simulink model "Inversores_simu"  (R2024b)
settings: Solver=FixedStepDiscrete  StartTime=0.0  StopTime=10/f  FixedStep=fixed_step  RelTol=1e-3
PostLoadFcn:
  | if any(exist('dsrtsu_mdlpostloadfcn', 'file') ~= 0), dsrtsu_mdlpostloadfcn('Execute', bdroot); end
InitFcn:
  | % Solver
  | fixed_step = 1e-6;
  | sample_time = fixed_step;
  | 
  | % Frecuencia fundamental del inversor
  | f = 60;
undefined symbols (not defined in the file): C
libraries: spsFourierLib x24, spsIGBTDiodeLib x8, spsMultimeterLib x4, spsRMSLib x4, spsTHDLib x4, spsSeriesRLCBranchLib x2, spsTriangleGeneratorLib x2, spsDCVoltageSourceLib x2, spsVoltageMeasurementLib x1, spspowerguiLib x1
settings Model: DSRTSU_INTERNAL_RTI_VER=530  DSRTSU_INTERNAL_RTI_TYPE=rti1202  RTICANMMDATA=struct('GeneralSetupData',struct('modelroot','C:\Users\jjmd2\OneDrive\Escritorio','generalsettings',struct('filesettings',struct('destfolder',struct('Name','RTICANMM_FILES','Check',1),'buildfolder',struct('Name','.','Check',1),'AbsDestfolder',struct('Name','C:\Users\jjmd2\OneDrive\Escritorio\RTICANMM_FILES'),'AbsBuildfolder',struct('Name','C:\Users\jjmd2\OneDrive\Escritorio'))),'options',struct('addpaths',1,'rmpaths',1,'addtrcexclusion',logical(1),'cannavigator',struct('checkmonitoring',0),'show_usrtrc',0,'use_usrtrc',0),'advanced',struct('options',ones(1,100)),'MPSetup',{{}},'RTI',struct('Type','RTI1202','Ver','7.11','Date','02-Nov-2018'),'modelname','libreria_potencia','block','libreria_potencia'))  Creator=jjmd2  LastModifiedBy=PC
settings SolverCC: AlgebraicLoopSolver=TrustRegion
settings OptimizationCC: BlockReduction=off
settings DebuggingCC: UnconnectedInputMsg=warning  UnconnectedOutputMsg=warning  UnconnectedLineMsg=warning
settings HardwareCC: ProdBitPerPointer=32  ProdBitPerSizeT=32  ProdBitPerPtrDiffT=32  ProdLargestAtomicInteger=Integer  ProdEndianess=BigEndian  ProdWordSize=32  ProdHWDeviceType=Custom Processor->Custom  TargetIntDivRoundTo=Zero  TargetEndianess=BigEndian  TargetHWDeviceType=Custom Processor->Custom
settings ModelReferenceCC: EnableRefExpFcnMdlSchedulingChecks=on
settings SFSimCC: MATLABDynamicMemAlloc=off
settings RTWCC: Description=dSPACE DS1202 Hardware Platform  SystemTargetFile=rti1202.tlc  MakeCommand=make_rti  TemplateMakefile=rti1202.tmf  GPUComputeCapability=3.5  DLArmComputeVersion=19.05
settings STFCustomTargetCC: ParMdlRefBuildCompliant=on  SystemTargetFile=rti1202.tlc
settings GRTTargetCC: TargetLangStandard=C89/C90 (ANSI)  CompOptLevelCompliant=off  ConcurrentExecutionCompliant=off  CombineOutputUpdateFcns=off  MatFileLogging=off  CPPClassGenCompliant=off  UseToolchainInfoCompliant=off

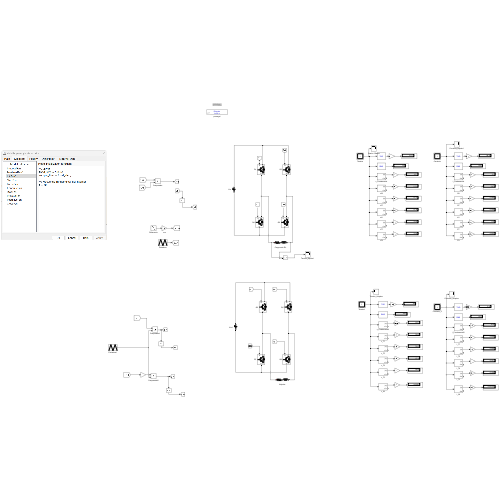
[thumbnail: Simulink's stored preview of the top-level diagram]
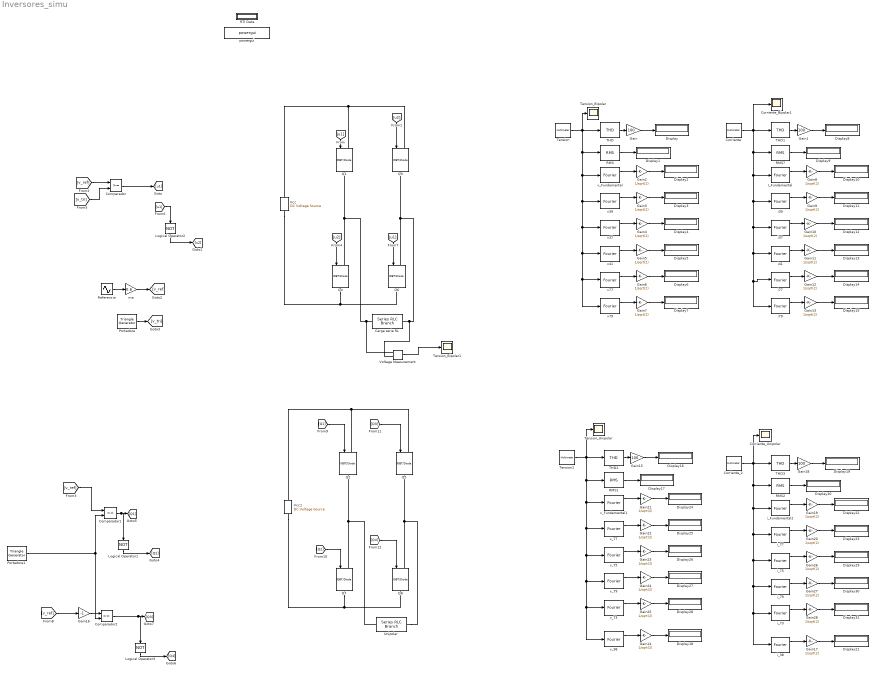
== system Inversores_simu ==
  Carga serie RL : spsSeriesRLCBranchLib/Series RLC Branch  LConnTagsString=__new0  RConnTagsString=__new0  BranchType=RL  Resistance=10  Inductance=5e-3  SetiL0=off  InitialCurrent=0  Capacitance=C  Setx0=off  InitialVoltage=0  Measurements=Branch voltage and current
  Comparador : RelationalOperator  OutDataTypeStr=boolean  RndMeth=Simplest  InputSameDT=off
  Comparador1 : RelationalOperator  OutDataTypeStr=boolean  RndMeth=Simplest  InputSameDT=off
  Comparador2 : RelationalOperator  OutDataTypeStr=boolean  RndMeth=Simplest  InputSameDT=off
  Corriente : spsMultimeterLib/Multimeter  L=4  sel=3  yselected={}  Gain=1  OutputType=Complex  PlotAtSimulationStop=off  PhasorSimulation=off
  Corriente_2 : spsMultimeterLib/Multimeter  L=4  sel=4  yselected={}  Gain=1  OutputType=Complex  PlotAtSimulationStop=off  PhasorSimulation=off
  Corriente_Bipolar1 : Scope
  Corriente_Unipolar : Scope
  Display{,1..31} (32 alike) : Display
  Gain{,1,15,18} (4 alike) : Gain  Gain=100
  Gain{2..14,17,19..28} (24 alike) : Gain  Gain=1/sqrt(2)
  Gain16 : Gain  Gain=-1
  I_Fundamental : spsFourierLib/Fourier  Freq=60  n=1  InInit=[0, 0]  Ts=sample_time
  Logical Operator1 : Logic  Operator=NOT  AllPortsSameDT=off  OutDataTypeStr=boolean
  Logical Operator2 : Logic  Operator=NOT  AllPortsSameDT=off  OutDataTypeStr=boolean
  Logical Operator3 : Logic  Operator=NOT  AllPortsSameDT=off  OutDataTypeStr=boolean
  Portadora : spsTriangleGeneratorLib/Triangle Generator  Freq=39*60  Phase=0  Ts=sample_time
  Portadora1 : spsTriangleGeneratorLib/Triangle Generator  Freq=38*60  Phase=0  Ts=sample_time
  Q{1..8} (8 alike) : spsIGBTDiodeLib/IGBT//Diode  Ron=1e-3  Rs=1000  Cs=0.1e-6  Measurements=off
  RMS{,1..2,7} (4 alike) : spsRMSLib/RMS  TrueRMS=on  Freq=60  RMSInit=120  Ts=sample_time
  RTI Data : Subsystem  Tag=struct('RTIDataServer',struct('RTIDataServerVs','2','RTIModelDescription','struct(''main'',''plantilla_modelos'',''sub'',''plantilla_modelos'',''isMp'',0)'))  LoadFcn="if exist('rtidc'), try,  rtidc('DataHostBlockClbLoad', gcbh); catch, disp(['Warning: ''LoadFcn'' for RTI Data block failed: ' lasterr]); end, end,"  mask(RTI_DATA_HOST){}
      mask help:
      | RTI Data Block.
      | This block is used by RTI to store internal model-dependent data.
      | Please keep this block on the root level of the model. Deleting this block will result in data loss.
      |
      | NEVER DELETE OR COPY THIS BLOCK!
      settings: CopyFcn="if exist('rtidc'), try,  rtidc('DataHostBlockClbCopy', gcbh); catch, disp(['Warning: ''CopyFcn'' for RTI Data block failed: ' lasterr]); end, end,"  DeleteFcn="if exist('rtidc'), try,  rtidc('DataHostBlockClbDelete', gcbh); catch, disp(['Warning: ''DeleteFcn'' for RTI Data block failed: ' lasterr]); end, end,"  ModelCloseFcn="if exist('rtidc'), try,  rtidc('DataHostBlockClbModelClose', gcbh); catch, disp(['Warning: ''ModelCloseFcn'' for RTI Data block failed: ' lasterr]); end, end,"  PreSaveFcn="if exist('rtidc'), try,  rtidc('DataHostBlockClbPreSave', gcbh); catch, disp(['Warning: ''PreSaveFcn'' for RTI Data block failed: ' lasterr]); end, end,"  PostSaveFcn="if exist('rtidc'), try,  rtidc('DataHostBlockClbPostSave', gcbh); catch, disp(['Warning: ''PostSaveFcn'' for RTI Data block failed: ' lasterr]); end, end,"  NameChangeFcn="if exist('rtidc'), try,  rtidc('DataHostBlockClbNameChange', gcbh); catch, disp(['Warning: ''NameChangeFcn'' for RTI Data block failed: ' lasterr]); end, end,"
      mask Help:
      | RTI Data Block.
      | This block is used by RTI to store internal model-dependent data.
      | Please keep this block on the root level of the model. Deleting this block will result in data loss.
      | 
      | NEVER DELETE OR COPY THIS BLOCK!
      mask Display:
      | text(0.5, 0.5, 'RTI Data', 'HorizontalAlignment', 'center');
      | plot([1 0]);
  Referencia : Sin  Frequency=2*pi*f  SampleTime=sample_time
  THD{,1..3} (4 alike) : spsTHDLib/THD  Freq=60  Ts=sample_time
  Tension : spsMultimeterLib/Multimeter  L=4  sel=1  yselected={}  Gain=1  OutputType=Complex  PlotAtSimulationStop=off  PhasorSimulation=off
  Tension1 : spsMultimeterLib/Multimeter  L=4  sel=2  yselected={}  Gain=1  OutputType=Complex  PlotAtSimulationStop=off  PhasorSimulation=off
  Tension_Bipolar : Scope
  Tension_Bipolar1 : Scope
  Tension_Unipolar : Scope
  Unipolar : spsSeriesRLCBranchLib/Series RLC Branch  LConnTagsString=__new0  RConnTagsString=__new0  BranchType=RL  Resistance=10  Inductance=5e-3  SetiL0=off  InitialCurrent=0  Capacitance=C  Setx0=off  InitialVoltage=0  Measurements=Branch voltage and current
  Vcc : spsDCVoltageSourceLib/DC Voltage Source  Amplitude=300  Measurements=None
  Vcc1 : spsDCVoltageSourceLib/DC Voltage Source  Amplitude=300  Measurements=None
  Voltage Measurement : spsVoltageMeasurementLib/Voltage Measurement  PhasorSimulation=off  OutputType=Complex  PSBequivalent=0
  i37 : spsFourierLib/Fourier  Freq=60  n=37  InInit=[0, 0]  Ts=sample_time
  i39 : spsFourierLib/Fourier  Freq=60  n=39  InInit=[0, 0]  Ts=sample_time
  i41 : spsFourierLib/Fourier  Freq=60  n=41  InInit=[0, 0]  Ts=sample_time
  i77 : spsFourierLib/Fourier  Freq=60  n=77  InInit=[0, 0]  Ts=sample_time
  i79 : spsFourierLib/Fourier  Freq=60  n=79  InInit=[0, 0]  Ts=sample_time
  i_38 : spsFourierLib/Fourier  Freq=60  n=38  InInit=[0, 0]  Ts=sample_time
  i_73 : spsFourierLib/Fourier  Freq=60  n=73  InInit=[0, 0]  Ts=sample_time
  i_75 : spsFourierLib/Fourier  Freq=60  n=75  InInit=[0, 0]  Ts=sample_time
  i_77 : spsFourierLib/Fourier  Freq=60  n=77  InInit=[0, 0]  Ts=sample_time
  i_79 : spsFourierLib/Fourier  Freq=60  n=79  InInit=[0, 0]  Ts=sample_time
  i_Fundamental2 : spsFourierLib/Fourier  Freq=60  n=1  InInit=[0, 0]  Ts=sample_time
  ma : Gain  Gain=0.6
  powergui : spspowerguiLib/powergui  Priority=1  SimulationMode=Discrete  SampleTime=sample_time  frequency=60  Iterations=50  frequencyindice=0  Pbase=100e6  ErrMax=1e-4  UnitsV=kV  UnitsW=MW  buscounter=0  FunctionMessages=off  echomessages=off  EnableUseOfTLC=off  CurrentSourceSwitches=off  DisableSnubberDevices=off  DisableRonSwitches=off  DisableVfSwitches=off  DisplayEquations=off  AutomaticDiscreteSolvers=off  SolverType=Tustin/Backward Euler (TBE)  Interpol=off  ExternalGateDelay=off  methode=off  Ts=100  x0status=blocks  SPID=off  SwTol=0  HookPort=off  NonlinearTolerance=1e-4  nMaxIteration=100  ContinueOnMaxIteration=off  RestoreLinks=warning  ResistiveCurrentMeasurement=off  Frange=[0:2:500]  Ylog=off  Xlog=on  ShowGrid=off  save=off  variable=ZData  structure=0  ZoomFFT=off  StartTime=0.0  cycles=1  DisplayStyle=1  fundamental=60  FreqAxis=off  MaxFrequency=1000  frequencyindicesteady=1  RmsSteady=1  display=off
  v37 : spsFourierLib/Fourier  Freq=60  n=37  InInit=[0, 0]  Ts=sample_time
  v39 : spsFourierLib/Fourier  Freq=60  n=39  InInit=[0, 0]  Ts=sample_time
  v41 : spsFourierLib/Fourier  Freq=60  n=41  InInit=[0, 0]  Ts=sample_time
  v77 : spsFourierLib/Fourier  Freq=60  n=77  InInit=[0, 0]  Ts=sample_time
  v79 : spsFourierLib/Fourier  Freq=60  n=79  InInit=[0, 0]  Ts=sample_time
  v_38 : spsFourierLib/Fourier  Freq=60  n=38  InInit=[0, 0]  Ts=sample_time
  v_73 : spsFourierLib/Fourier  Freq=60  n=73  InInit=[0, 0]  Ts=sample_time
  v_75 : spsFourierLib/Fourier  Freq=60  n=75  InInit=[0, 0]  Ts=sample_time
  v_77 : spsFourierLib/Fourier  Freq=60  n=77  InInit=[0, 0]  Ts=sample_time
  v_79 : spsFourierLib/Fourier  Freq=60  n=79  InInit=[0, 0]  Ts=sample_time
  v_Fundamental : spsFourierLib/Fourier  Freq=60  n=1  InInit=[0, 0]  Ts=sample_time
  v_Fundamental1 : spsFourierLib/Fourier  Freq=60  n=1  InInit=[0, 0]  Ts=sample_time
  wires:
  ma/1 -> [v_ref]
  Referencia/1 -> ma/1
  THD/1 -> Gain/1
  [u2] -> Q3/1
  Comparador/1 -> [u1]
  Portadora/1 -> [v_tri]
  [u2] -> Q4/1
  Logical Operator2/1 -> [u2]
  [u1] -> Q1/1
  [v_ref] -> Comparador/1
  [v_tri] -> Comparador/2
  Gain/1 -> Display/1
  RMS/1 -> Display1/1
  Tension/1 -> Tension_Bipolar/1, v_Fundamental/1, v37/1, v41/1, v77/1, v79/1, v39/1, RMS/1, THD/1
  [u1] -> Logical Operator2/1
  [u1] -> Q6/1
  v_Fundamental/1 -> Gain2/1
  v39/1 -> Gain3/1
  v37/1 -> Gain4/1
  v41/1 -> Gain5/1
  v77/1 -> Gain6/1
  v79/1 -> Gain7/1
  Gain7/1 -> Display7/1
  Gain6/1 -> Display6/1
  Gain5/1 -> Display5/1
  Gain4/1 -> Display4/1
  Gain3/1 -> Display3/1
  Gain2/1 -> Display2/1
  Gain8/1 -> Display10/1
  Gain9/1 -> Display11/1
  Gain10/1 -> Display12/1
  Gain11/1 -> Display13/1
  Gain12/1 -> Display14/1
  Gain13/1 -> Display15/1
  i79/1 -> Gain13/1
  i77/1 -> Gain12/1
  i41/1 -> Gain11/1
  i37/1 -> Gain10/1
  i39/1 -> Gain9/1
  I_Fundamental/1 -> Gain8/1
  Corriente/1 -> Corriente_Bipolar1/1, THD1/1, RMS7/1, i39/1, i41/1, i77/1, i79/1, i37/1, I_Fundamental/1
  RMS7/1 -> Display9/1
  Gain1/1 -> Display8/1
  THD1/1 -> Gain1/1
  [Q4] -> Q8/1
  [Q1] -> Q2/1
  Portadora1/1 -> Comparador1/2, Comparador2/2
  Gain21/1 -> Display24/1
  Gain22/1 -> Display25/1
  Gain23/1 -> Display26/1
  Gain24/1 -> Display27/1
  Gain25/1 -> Display28/1
  v_73/1 -> Gain25/1
  v_79/1 -> Gain24/1
  v_75/1 -> Gain23/1
  v_77/1 -> Gain22/1
  v_Fundamental1/1 -> Gain21/1
  Tension1/1 -> THD2/1, RMS1/1, v_77/1, v_38/1, v_73/1, v_79/1, v_75/1, v_Fundamental1/1, Tension_Unipolar/1
  RMS1/1 -> Display17/1
  Gain15/1 -> Display16/1
  THD2/1 -> Gain15/1
  v_38/1 -> Gain14/1
  Gain14/1 -> Display18/1
  [v_ref] -> Gain16/1
  Gain16/1 -> Comparador2/1
  [v_ref] -> Comparador1/1
  Comparador1/1 -> Logical Operator1/1, [Q1]
  Logical Operator1/1 -> [Q2]
  Logical Operator3/1 -> [Q4]
  Comparador2/1 -> [Q3], Logical Operator3/1
  [Q2] -> Q7/1
  [Q3] -> Q5/1
  Gain17/1 -> Display21/1
  i_38/1 -> Gain17/1
  THD3/1 -> Gain18/1
  Gain18/1 -> Display19/1
  RMS2/1 -> Display20/1
  Corriente_2/1 -> Corriente_Unipolar/1, i_Fundamental2/1, i_75/1, i_79/1, i_73/1, i_38/1, i_77/1, RMS2/1, THD3/1
  i_Fundamental2/1 -> Gain19/1
  i_77/1 -> Gain20/1
  i_75/1 -> Gain26/1
  i_79/1 -> Gain27/1
  i_73/1 -> Gain28/1
  Gain28/1 -> Display31/1
  Gain27/1 -> Display30/1
  Gain26/1 -> Display29/1
  Gain20/1 -> Display23/1
  Gain19/1 -> Display22/1
  Voltage Measurement/1 -> Tension_Bipolar1/1
  connections:
  Q4/LConn1 -- Voltage Measurement/LConn1 -- Carga serie RL/LConn1 -- Q1/RConn1
  Q1/LConn1 -- Vcc/RConn1 -- Q3/LConn1
  Q4/RConn1 -- Vcc/LConn1 -- Q6/RConn1
  Q6/LConn1 -- Voltage Measurement/LConn2 -- Carga serie RL/RConn1 -- Q3/RConn1
  Q2/RConn1 -- Q7/LConn1 -- Unipolar/LConn1
  Vcc1/RConn1 -- Q2/LConn1 -- Q5/LConn1
  Vcc1/LConn1 -- Q7/RConn1 -- Q8/RConn1
  Q5/RConn1 -- Q8/LConn1 -- Unipolar/RConn1

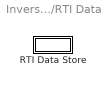
== system Inversores_simu/RTI Data ==
  RTI Data Store : Subsystem  Tag="struct('private',struct('version',struct('dsVer',uint32(2),'dsVerCreation',uint32(2),'RTI',struct('ver','7.11','type','RTI1202')),'access',struct('type','Model','isPerm',1,'created',['03-Jun-2021 09:00:50'],'modified',['12-Mar-2024 20:44:21'],'location','')),'public',struct('main',struct('data',[]),'sub',struct('name',{{'plantilla_modelos'}},'data',{{struct('TH',struct('thTaskInfo',struct('taskType',{'TIMER','HWINT','TMRINT','SWINT','GLINT'},'tasksNumOf',{1,0,0,0,0},'srcIds',{{'TIMERA'},{},{},{},{}},'taskNames',{{['Timer Task 1']},{},{},{},{}})),'th_tc',struct('dataType','TASK','taskGroupId','','taskGroupList',{{}},'taskSchedulingPolicy','FCFS','taskType','TIMER','blkh',-1,'srcId','TIMERA','srcSgnName',['Timer A interrupt'],'srcCpuName','','taskName',['Timer Task 1  [0.0001] s'],'taskNameDisplayExt','','smplTime',0.0001,'smplTimeOffs',0,'hasFixedPriority',0,'priority',1,'hasFixedOvc',0,'ovcType',1,'ovcMax',1),'tc_th',struct('dataType','TASK','taskGroupId','','taskGroupList',{{}},'taskSchedulingPolicy','FCFS','taskType','TIMER','blkh',-1,'srcId','TIMERA','srcSgnName',['Timer A interrupt'],'srcCpuName','','taskName',['Timer Task 1  [0.0001] s'],'taskNameDisplayExt','','smplTime',0.0001,'smplTimeOffs',0,'hasFixedPriority',0,'priority',1,'hasFixedOvc',0,'ovcType',1,'ovcMax',1))}})))"  mask(RTI_DATA_STORE){}
      mask help:
      | RTI Data Store Block. This block is used by RTI to store internal model dependent data. Deleting this block will result in data loss.
      |
      | NEVER DELETE, COPY, OR MODIFY THIS BLOCK!
      mask Help:
      | RTI Data Store Block. This block is used by RTI to store internal model dependent data. Deleting this block will result in data loss.
      | 
      | NEVER DELETE, COPY, OR MODIFY THIS BLOCK!
      mask Display: text(0.5, 0.5, ' ', 'HorizontalAlignment', 'center');

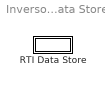
== system Inversores_simu/RTI Data/RTI Data Store ==
  RTI Data Store : Subsystem  mask(RTI_DATA_STORE){}
      mask help:
      | RTI Data Store Block. This block is used by RTI to store internal model dependent data. Deleting this block will result in data loss.
      |
      | NEVER DELETE, COPY, OR MODIFY THIS BLOCK!
      mask Help:
      | RTI Data Store Block. This block is used by RTI to store internal model dependent data. Deleting this block will result in data loss.
      | 
      | NEVER DELETE, COPY, OR MODIFY THIS BLOCK!
      mask Display: text(0.5, 0.5, ' ', 'HorizontalAlignment', 'center');

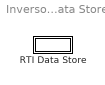
== system Inversores_simu/RTI Data/RTI Data Store/RTI Data Store ==
  RTI Data Store : Subsystem  mask(RTI_DATA_STORE){}
      mask help:
      | RTI Data Store Block. This block is used by RTI to store internal model dependent data. Deleting this block will result in data loss.
      |
      | NEVER DELETE, COPY, OR MODIFY THIS BLOCK!
      mask Help:
      | RTI Data Store Block. This block is used by RTI to store internal model dependent data. Deleting this block will result in data loss.
      | 
      | NEVER DELETE, COPY, OR MODIFY THIS BLOCK!
      mask Display: text(0.5, 0.5, ' ', 'HorizontalAlignment', 'center');

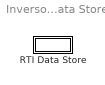
== system Inversores_simu/RTI Data/RTI Data Store/RTI Data Store/RTI Data Store ==
  RTI Data Store : Subsystem  mask(RTI_DATA_STORE){}
      mask help:
      | RTI Data Store Block. This block is used by RTI to store internal model dependent data. Deleting this block will result in data loss.
      |
      | NEVER DELETE, COPY, OR MODIFY THIS BLOCK!
      mask Help:
      | RTI Data Store Block. This block is used by RTI to store internal model dependent data. Deleting this block will result in data loss.
      | 
      | NEVER DELETE, COPY, OR MODIFY THIS BLOCK!
      mask Display: text(0.5, 0.5, ' ', 'HorizontalAlignment', 'center');

== system Inversores_simu/RTI Data/RTI Data Store/RTI Data Store/RTI Data Store/RTI Data Store ==
